simulink model "SurgeSpeed"  (R2015b)
settings: Solver=ode45  StartTime=tstart  StopTime=tstop  RelTol=1e-3
values from neighbouring files (symbols this model uses):
  c = 0    [AnalyseSurgeSpeed.m]    (also in SurgeDynamicsTest.m; SurgeSpeedTest.m; analyse_dynamics.m; analyse_sway_dynamics.m)
  delta_dot_max = deg2rad(0.4)    [SurgeSpeedTest.m]    (also in Yaw and Yaw-rate controller.mat = 0.00698131700798; run_task1_8.m)
  delta_max = deg2rad(25)    [SurgeSpeedTest.m]    (also in Yaw and Yaw-rate controller.mat = 0.436332312999; msfartoystyring.m = 0.436332312999; run_task1_8.m)
  k_b0 = 0.009    [SurgeSpeedTest.m]    (also in Yaw and Yaw-rate controller.mat; run_task1_8.m)
  k_b1 = b_2(2)    [SurgeSpeedTest.m]    (also in Yaw and Yaw-rate controller.mat = 3.06871796591e-14; run_task1_8.m)
  k_b2 = b_2(3)    [SurgeSpeedTest.m]    (also in Yaw and Yaw-rate controller.mat = 291.893339409; run_task1_8.m)
  k_b3 = b_2(1)    [SurgeSpeedTest.m]    (also in Yaw and Yaw-rate controller.mat = 1233422.7042; run_task1_8.m)
  kd_psi = 3    [SurgeSpeedTest.m]    (also in Yaw and Yaw-rate controller.mat; run_task1_8.m)
  kd_r = 5e3    (= 5000)    [SurgeSpeedTest.m]    (also in Yaw and Yaw-rate controller.mat; run_task1_8.m)
  ki_psi = 2e-5    (= 2e-05)    [SurgeSpeedTest.m]    (also in Yaw and Yaw-rate controller.mat; run_task1_8.m)
  ki_r = 1/3    (= 0.333333333333)    [SurgeSpeedTest.m]    (also in Yaw and Yaw-rate controller.mat; run_task1_8.m)
  kp_psi = 15e-3    (= 0.015)    [SurgeSpeedTest.m]    (also in Yaw and Yaw-rate controller.mat; run_task1_8.m)
  kp_r = 300    [SurgeSpeedTest.m]    (also in Yaw and Yaw-rate controller.mat; run_task1_8.m)
  n_c = elm    [AnalyseSurgeSpeed.m]    (also in SurgeDynamicsTest.m = nc_list(i); SurgeSpeedTest.m = nc_list(i); analyse_dynamics.m = nc_list(i); matlab.mat = 8.9)
  N_psi = deg2rad(1)    [SurgeSpeedTest.m]    (also in Yaw and Yaw-rate controller.mat = 0.0174532925199; run_task1_8.m)
  N_r = deg2rad(0.8)    [SurgeSpeedTest.m]    (also in Yaw and Yaw-rate controller.mat = 0.013962634016; run_task1_8.m)
  psi0 = 0    [AnalyseSurgeSpeed.m]    (also in SurgeDynamicsTest.m; SurgeSpeedTest.m; analyse_dynamics.m; analyse_sway_dynamics.m)
  r0 = 0    [AnalyseSurgeSpeed.m]    (also in SurgeDynamicsTest.m; SurgeSpeedTest.m; analyse_dynamics.m; analyse_sway_dynamics.m)
  r_max = deg2rad(0.35)    [SurgeSpeedTest.m]    (also in Yaw and Yaw-rate controller.mat = 0.00610865238198; run_task1_8.m)
  tsamp = 10    [AnalyseSpeedCharacteristis.m]    (also in AnalyseSpeedModel.m; AnalyseSurgeSpeed.m; Analyse_steadystate.m; SurgeDynamicsTest.m)
  v0 = [0.00001 0]'    [AnalyseSurgeSpeed.m]    (also in SurgeDynamicsTest.m = [1e-7 0]'; SurgeSpeedTest.m = [1e-7 0]'; analyse_dynamics.m = [1e-7 0]'; analyse_sway_dynamics.m = [6.63 0]')
  w_psi = 0.04    [SurgeSpeedTest.m]    (also in Yaw and Yaw-rate controller.mat; run_task1_8.m = deg2rad(0.2))
  w_r = deg2rad(0.3)    [SurgeSpeedTest.m]    (also in Yaw and Yaw-rate controller.mat = 0.00523598775598; run_task1_8.m)
undefined symbols (not defined in the file or in its folder): msfartoystyring
undefined symbols (not defined in the file): p0
libraries: simulink x2
settings Model: ExtModeAutoUpdateStatusClock=off  Creator=christh  LastModifiedBy=Erik
settings DataIOCC: SaveFormat=Array  SignalLoggingSaveFormat=ModelDataLogs
settings OptimizationCC: ExpressionDepthLimit=2147483647  InitFltsAndDblsToZero=on
settings DebuggingCC: UnderspecifiedInitializationDetection=Classic  MergeDetectMultiDrivingBlocksExec=none  SolverPrmCheckMsg=warning  FcnCallInpInsideContextMsg=UseLocalSettings  StateNameClashWarn=warning
settings HardwareCC: ProdBitPerPointer=32  ProdLargestAtomicFloat=None  ProdIntDivRoundTo=Undefined  ProdEndianess=Unspecified  ProdWordSize=32  ProdHWDeviceType=32-bit Generic
settings GRTTargetCC: GeneratePreprocessorConditionals=Disable all  CombineOutputUpdateFcns=off  GRTInterface=on
settings ConfigComp: CovModelRefEnable=Off

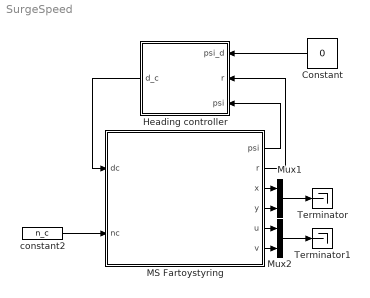
== system SurgeSpeed ==
  Constant : Constant  Value=0
  Heading controller : Subsystem
  MS Fartoystyring : Subsystem  mask(MS Fartoystyring for Assignment 3 G&C){x0=p0(1), y0=p0(2), u0=v0(1), v0=v0(2), psi0=psi0, r0=r0, c=c}
      mask prompts: x0 "x(t0) (m)"; y0 "y(t0) (m)"; u0 "u(t0) (m/s)"; v0 "v(t0) (m/s)"; psi0 "psi(t0) (rad)"; r0 "r(t0) (rad/s)"; c "current (0 or 1)"
      mask help:
      | Block corresponding to Figure 1 in the assignment text. Gives the response of the ship.
      |
      | The design speed of MS Fartoystyring is u=8.23 m/s.
      |
      | Input:
      | dc: commanded rudder (rad), dmax=25*pi/180
      | nc: commanded shaft speed (rad/s), nmax=85*2*pi/60
      |
      | Output:
      | x: north pos (m)
      | y: east pos (m)
      | u: surge (m/s)
      | v: sway (m/s)
      | psi: heading (rad)
      | r: yaw (rad/s)
      mask Help: Comments, bugs and help requests can be directed to the TA. Email on course website.
  Mux1 : Mux  Inputs=2
  Mux2 : Mux  Inputs=2
  Terminator : Terminator
  Terminator1 : Terminator
  constant2 : Constant  Value=n_c
  wires:
  MS Fartoystyring/1(psi) -> Heading controller/3(psi)
  MS Fartoystyring/2(r) -> Heading controller/2(r)
  MS Fartoystyring/3(x) -> Mux1/1
  MS Fartoystyring/4(y) -> Mux1/2
  Mux1/1 -> Terminator/1
  Constant/1 -> Heading controller/1(psi_d)
  Heading controller/1(d_c) -> MS Fartoystyring/1(dc)
  MS Fartoystyring/6(v) -> Mux2/2
  MS Fartoystyring/5(u) -> Mux2/1
  Mux2/1 -> Terminator1/1
  constant2/1 -> MS Fartoystyring/2(nc)

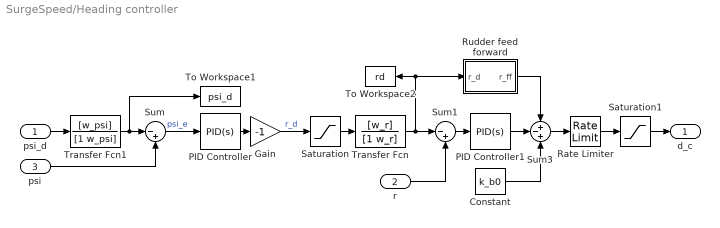
== system SurgeSpeed/Heading controller ==
  psi_d : Inport
  r : Inport  Port=2
  psi : Inport  Port=3
  Constant : Constant  Value=k_b0
  Gain : Gain  Gain=-1
  PID Controller : simulink/Continuous/PID Controller  Controller=PID  TimeDomain=Continuous-time  SampleTime=-1  IntegratorMethod=Forward Euler  FilterMethod=Forward Euler  Form=Parallel  UseFilter=on  ControllerParametersSource=internal  P=kp_psi  I=ki_psi  D=kd_psi  N=N_psi  InitialConditionSource=internal  InitialConditionForIntegrator=0  InitialConditionForFilter=0  ExternalReset=none  LimitOutput=off  UpperSaturationLimit=inf  LowerSaturationLimit=-inf  LinearizeAsGain=on  AntiWindupMode=none  Kb=1  TrackingMode=off  Kt=1  PParamMin=[]  PParamMax=[]  IParamMin=[]  IParamMax=[]  DParamMin=[]  DParamMax=[]  NParamMin=[]  NParamMax=[]  KbParamMin=[]  KbParamMax=[]  KtParamMin=[]  KtParamMax=[]  POutMin=[]  POutMax=[]  IOutMin=[]  IOutMax=[]  DOutMin=[]  DOutMax=[]  NOutMin=[]  NOutMax=[]  KbOutMin=[]  KbOutMax=[]  KtOutMin=[]  KtOutMax=[]  IntegratorOutMin=[]  IntegratorOutMax=[]  FilterOutMin=[]  FilterOutMax=[]  SumOutMin=[]  SumOutMax=[]  SumI1OutMin=[]  SumI1OutMax=[]  SumI2OutMin=[]  SumI2OutMax=[]  SumI3OutMin=[]  SumI3OutMax=[]  SumDOutMin=[]  SumDOutMax=[]  SaturationOutMin=[]  SaturationOutMax=[]  IntegratorContinuousStateAttributes=''  IntegratorStateMustResolveToSignalObject=off  IntegratorRTWStateStorageClass=Auto  FilterContinuousStateAttributes=''  FilterStateMustResolveToSignalObject=off  FilterRTWStateStorageClass=Auto  DifferentiatorICPrevScaledInput=0  DifferentiatorOutMin=[]  DifferentiatorOutMax=[]
  PID Controller1 : simulink/Continuous/PID Controller  Controller=PID  TimeDomain=Continuous-time  SampleTime=-1  IntegratorMethod=Forward Euler  FilterMethod=Forward Euler  Form=Parallel  UseFilter=on  ControllerParametersSource=internal  P=kp_r  I=ki_r  D=kd_r  N=N_r  InitialConditionSource=internal  InitialConditionForIntegrator=0  InitialConditionForFilter=0  ExternalReset=none  LimitOutput=off  UpperSaturationLimit=inf  LowerSaturationLimit=-inf  LinearizeAsGain=on  AntiWindupMode=none  Kb=1  TrackingMode=off  Kt=1  PParamMin=[]  PParamMax=[]  IParamMin=[]  IParamMax=[]  DParamMin=[]  DParamMax=[]  NParamMin=[]  NParamMax=[]  KbParamMin=[]  KbParamMax=[]  KtParamMin=[]  KtParamMax=[]  POutMin=[]  POutMax=[]  IOutMin=[]  IOutMax=[]  DOutMin=[]  DOutMax=[]  NOutMin=[]  NOutMax=[]  KbOutMin=[]  KbOutMax=[]  KtOutMin=[]  KtOutMax=[]  IntegratorOutMin=[]  IntegratorOutMax=[]  FilterOutMin=[]  FilterOutMax=[]  SumOutMin=[]  SumOutMax=[]  SumI1OutMin=[]  SumI1OutMax=[]  SumI2OutMin=[]  SumI2OutMax=[]  SumI3OutMin=[]  SumI3OutMax=[]  SumDOutMin=[]  SumDOutMax=[]  SaturationOutMin=[]  SaturationOutMax=[]  IntegratorContinuousStateAttributes=''  IntegratorStateMustResolveToSignalObject=off  IntegratorRTWStateStorageClass=Auto  FilterContinuousStateAttributes=''  FilterStateMustResolveToSignalObject=off  FilterRTWStateStorageClass=Auto  DifferentiatorICPrevScaledInput=0  DifferentiatorOutMin=[]  DifferentiatorOutMax=[]
  Rate Limiter : RateLimiter  RisingSlewLimit=delta_dot_max  FallingSlewLimit=-delta_dot_max  SampleTimeMode=inherited
  Rudder feed forward : Subsystem
  Saturation : Saturate  UpperLimit=r_max  LowerLimit=-r_max
  Saturation1 : Saturate  UpperLimit=delta_max  LowerLimit=-delta_max
  Sum : Sum  Inputs=|-+
  Sum1 : Sum  Inputs=|-+
  Sum3 : Sum  Inputs=+-+
  To Workspace1 : ToWorkspace  VariableName=psi_d  SampleTime=tsamp
  To Workspace2 : ToWorkspace  VariableName=rd  SampleTime=tsamp
  Transfer Fcn : TransferFcn  Numerator=[w_r]  Denominator=[1 w_r]
  Transfer Fcn1 : TransferFcn  Numerator=[w_psi]  Denominator=[1 w_psi]
  d_c : Outport
  wires:
  Sum/1 -> PID Controller/1  "psi_e"
  psi_d/1 -> Transfer Fcn1/1
  psi/1 -> Sum/2
  Rate Limiter/1 -> Saturation1/1
  Constant/1 -> Sum3/3
  Saturation/1 -> Transfer Fcn/1
  Transfer Fcn/1 -> Sum1/1, Rudder feed forward/1(r_d), To Workspace2/1
  Sum3/1 -> Rate Limiter/1
  PID Controller1/1 -> Sum3/2
  Sum1/1 -> PID Controller1/1
  r/1 -> Sum1/2
  Saturation1/1 -> d_c/1
  PID Controller/1 -> Gain/1
  Rudder feed forward/1(r_ff) -> Sum3/1
  Transfer Fcn1/1 -> To Workspace1/1, Sum/1
  Gain/1 -> Saturation/1  "r_d"

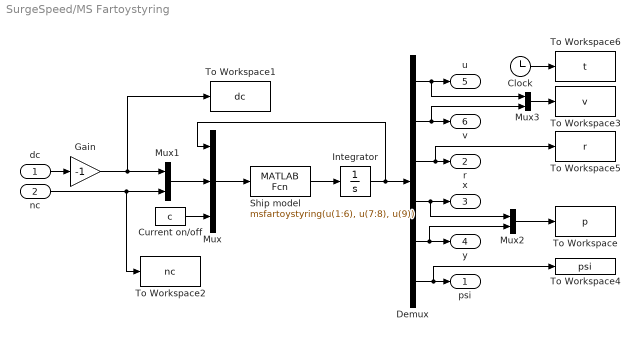
== system SurgeSpeed/MS Fartoystyring ==
  dc : Inport
  nc : Inport  Port=2
  Clock : Clock
  Current on/off : Constant  Value=c
  Demux : Demux  Outputs=6
  Gain : Gain  Gain=-1
  Integrator : Integrator  InitialCondition=[u0 v0 r0 x0 y0 psi0]'
  Mux : Mux  Inputs=3
  Mux1 : Mux  Inputs=2
  Mux2 : Mux  Inputs=2
  Mux3 : Mux  Inputs=2
  Ship model : MATLABFcn  MATLABFcn=msfartoystyring(u(1:6), u(7:8), u(9))  OutputDimensions=6
  To Workspace : ToWorkspace  VariableName=p  SampleTime=tsamp
  To Workspace1 : ToWorkspace  VariableName=dc  SampleTime=tsamp
  To Workspace2 : ToWorkspace  VariableName=nc  SampleTime=tsamp
  To Workspace3 : ToWorkspace  VariableName=v  SampleTime=tsamp
  To Workspace4 : ToWorkspace  VariableName=psi  SampleTime=tsamp
  To Workspace5 : ToWorkspace  VariableName=r  SampleTime=tsamp
  To Workspace6 : ToWorkspace  VariableName=t  SampleTime=tsamp
  psi : Outport
  r : Outport  Port=2
  x : Outport  Port=3
  y : Outport  Port=4
  u : Outport  Port=5
  v : Outport  Port=6
  wires:
  Integrator/1 -> Mux/1, Demux/1
  Mux1/1 -> Mux/2
  dc/1 -> Gain/1
  nc/1 -> Mux1/2, To Workspace2/1
  Demux/1 -> Mux3/1, u/1
  Demux/2 -> Mux3/2, v/1
  Demux/3 -> To Workspace5/1, r/1
  Demux/4 -> Mux2/1, x/1
  Demux/5 -> y/1, Mux2/2
  Demux/6 -> To Workspace4/1, psi/1
  Current on/off/1 -> Mux/3
  Ship model/1 -> Integrator/1
  Mux/1 -> Ship model/1
  Mux2/1 -> To Workspace/1
  Clock/1 -> To Workspace6/1
  Mux3/1 -> To Workspace3/1
  Gain/1 -> To Workspace1/1, Mux1/1

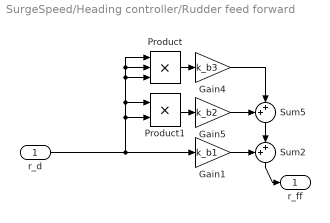
== system SurgeSpeed/Heading controller/Rudder feed forward ==
  r_d : Inport
  Gain1 : Gain  Gain=k_b1
  Gain4 : Gain  Gain=k_b3
  Gain5 : Gain  Gain=k_b2
  Product : Product  Inputs=3
  Product1 : Product
  Sum2 : Sum  Inputs=++|
  Sum5 : Sum  Inputs=++|
  r_ff : Outport
  wires:
  Gain4/1 -> Sum5/2
  Sum5/1 -> Sum2/2
  r_d/1 -> Product1/2, Product1/1, Product/1, Product/2, Product/3, Gain1/1
  Gain5/1 -> Sum5/1
  Product/1 -> Gain4/1
  Gain1/1 -> Sum2/1
  Product1/1 -> Gain5/1
  Sum2/1 -> r_ff/1
